simulink model "sub_model_first_gear"  (R2020b)
settings: Solver=VariableStepAuto  StartTime=0.0  StopTime=10.0  RelTol=1e-3
settings Model: Creator=morro  LastModifiedBy=morro

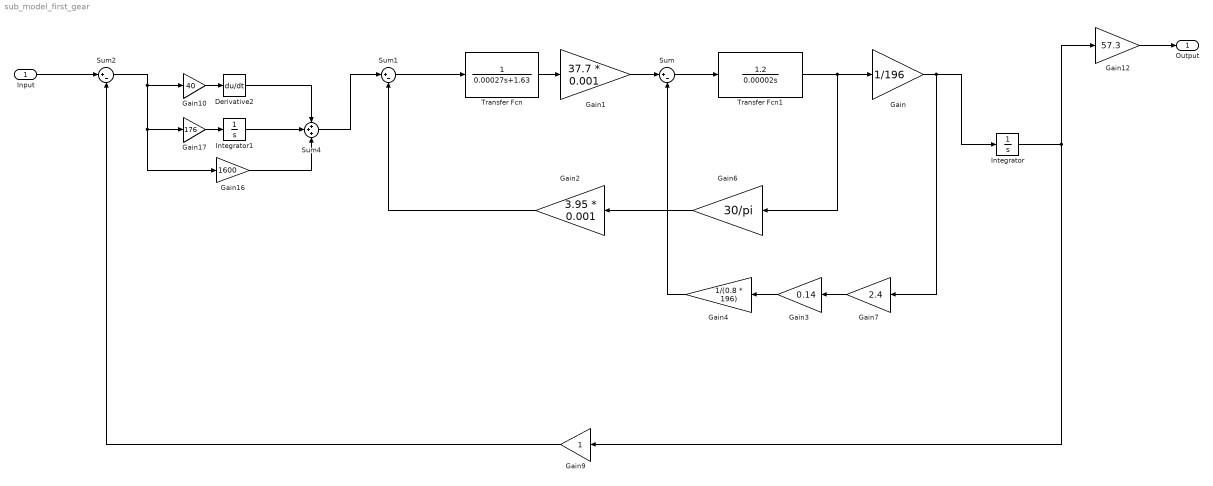
== system sub_model_first_gear ==
  Input : Inport
  Derivative2 : Derivative
  Gain : Gain  Gain=1/196
  Gain1 : Gain  Gain=37.7 * 0.001
  Gain10 : Gain  Gain=40
  Gain12 : Gain  Gain=57.3
  Gain16 : Gain  Gain=1600
  Gain17 : Gain  Gain=176
  Gain2 : Gain  Gain=3.95 * 0.001
  Gain3 : Gain  Gain=0.14
  Gain4 : Gain  Gain=1/(0.8 * 196)
  Gain6 : Gain  Gain=30/pi
  Gain7 : Gain  Gain=2.4
  Gain9 : Gain
  Integrator : Integrator  InitialCondition=1e-7
  Integrator1 : Integrator  InitialCondition=1e-7
  Sum : Sum  Inputs=|+-
  Sum1 : Sum  Inputs=|+-
  Sum2 : Sum  Inputs=|+-
  Sum4 : Sum  Inputs=+++
  Transfer Fcn : TransferFcn  Denominator=[0.00027 1.63]
  Transfer Fcn1 : TransferFcn  Numerator=[1.2]  Denominator=[0.00002 0]
  Output : Outport
  wires:
  Sum4/1 -> Sum1/1
  Derivative2/1 -> Sum4/1
  Sum1/1 -> Transfer Fcn/1
  Sum2/1 -> Gain16/1, Gain17/1, Gain10/1
  Gain7/1 -> Gain3/1
  Sum/1 -> Transfer Fcn1/1
  Integrator1/1 -> Sum4/2
  Gain6/1 -> Gain2/1
  Gain10/1 -> Derivative2/1
  Transfer Fcn1/1 -> Gain6/1, Gain/1
  Gain16/1 -> Sum4/3
  Input/1 -> Sum2/1
  Gain17/1 -> Integrator1/1
  Gain3/1 -> Gain4/1
  Gain/1 -> Gain7/1, Integrator/1
  Gain9/1 -> Sum2/2
  Gain2/1 -> Sum1/2
  Integrator/1 -> Gain9/1, Gain12/1
  Transfer Fcn/1 -> Gain1/1
  Gain1/1 -> Sum/1
  Gain4/1 -> Sum/2
  Gain12/1 -> Output/1
